simulink model "threeDiskOscillatorRig_Q2_3_v2"  (R2020a)
settings: Solver=VariableStepAuto  StartTime=0.0  StopTime=simTime  RelTol=1e-8
values from neighbouring files (symbols this model uses):
  atan_scale = 100    [ECP_values_final.mat]    (also in Q2-5.mat; Residual_generators.mat; Residual_generatorsQ2.mat; threeDiskOscillator_ALL.m)
  b_1 = 0.00287081256979    [ECP_values_final.mat]    (also in Q2-5.mat; Residual_generators.mat; Residual_generatorsQ2.mat; threeDiskOscillator_ALL.m = mean(ECP_values([6 7])))
  b_2 = 0.000164101446955    [ECP_values_final.mat]    (also in Q2-5.mat; Residual_generators.mat; Residual_generatorsQ2.mat; threeDiskOscillator_ALL.m = mean(ECP_values([8 9])))
  b_3 = 0.000179179608867    [ECP_values_final.mat]    (also in Q2-5.mat; Residual_generators.mat; Residual_generatorsQ2.mat; threeDiskOscillator_ALL.m = mean(ECP_values([10 11])))
  B_change = [1  0; 0  0]    [ECP_values_final.mat]    (also in Q2-5.mat; Residual_generators.mat; Residual_generatorsQ2.mat; threeDiskOscillator_ALL.m = [1 0;0 0])
  C = [1 0 0 0 0 0 0 1 0 0 0 0 ... (18 elements, 3x6)]    [ECP_values_final.mat]    (also in Q2-5.mat; Residual_generators.mat; Residual_generatorsQ2.mat; threeDiskOscillator_ALL.m = double(jacobian(g, x)))
  C_aug = [1 0 0 0 0 0 0 1 0 0 0 0 ... (21 elements, 3x7)]    [ECP_values_final.mat]    (also in Q2-5.mat; Residual_generators.mat; Residual_generatorsQ2.mat; threeDiskOscillator_ALL.m = [C zeros(3, 1)])
  den1 =     [ECP_values_final.mat]    (also in Q2-5.mat; Residual_generators.mat; Residual_generatorsQ2.mat)
  den2 =     [ECP_values_final.mat]    (also in Q2-5.mat; Residual_generators.mat; Residual_generatorsQ2.mat)
  detect_time = 45    [ECP_values_final.mat]    (also in Q2-5.mat = 28.75; Residual_generators.mat = 28.75; Residual_generatorsQ2.mat = 28.75; threeDiskOscillator_ALL.m = 28.75)
  F_aug = [0.990702939697 -4.62811632173 0.0121231655 6.0271208888 2.24543739426e-05 0.0224199828886 0 0.00397798624468 0.985916806084 1.6181632514e-05 0.0121036964897 1.79648757592e-08 ... (49 elements, 7x7)]    [ECP_values_final.mat]    (also in Q2-5.mat; Residual_generators.mat; Residual_generatorsQ2.mat; threeDiskOscillator_ALL.m = [F_d E)
  f_m = [0 -0.025 0]    [ECP_values_final.mat]    (also in Q2-5.mat; Residual_generators.mat; Residual_generatorsQ2.mat; threeDiskOscillator_ALL.m = [0;-0.025;0])
  f_m_time = 8.5    [ECP_values_final.mat]    (also in Q2-5.mat; Residual_generators.mat; Residual_generatorsQ2.mat; threeDiskOscillator_ALL.m)
  f_u = [0 0]    [ECP_values_final.mat]    (also in Q2-5.mat; Residual_generators.mat; Residual_generatorsQ2.mat; threeDiskOscillator_ALL.m = [0;0])
  f_u_time = 25    [ECP_values_final.mat]    (also in Q2-5.mat; Residual_generators.mat; Residual_generatorsQ2.mat; threeDiskOscillator_ALL.m)
  G_aug = [0.00334221577476 1.66717035551 6.79109721451e-06 0.00678170721861 5.02271998836e-09 7.52906281318e-06 0 6.79109721451e-06 0.00678170721861 0.00435611271714 2.16907893788 8.06078126345e-06 ... (14 elements, 7x2)]    [ECP_values_final.mat]    (also in Q2-5.mat; Residual_generators.mat; Residual_generatorsQ2.mat; threeDiskOscillator_ALL.m = [G_d; zeros(1, 2)])
  h = 7.56835261331    [ECP_values_final.mat]    (also in Q2-5.mat; Residual_generators.mat = 0; Residual_generatorsQ2.mat = 0; threeDiskOscillator_ALL.m = chi2inv(1 - P_F, 1)/2)
  J_1 = 0.00238607064451    [ECP_values_final.mat]    (also in Q2-5.mat; Residual_generators.mat; Residual_generatorsQ2.mat; threeDiskOscillator_ALL.m = ECP_values(1))
  J_2 = 0.00182883419357    [ECP_values_final.mat]    (also in Q2-5.mat; Residual_generators.mat; Residual_generatorsQ2.mat; threeDiskOscillator_ALL.m = ECP_values(2))
  J_3 = 0.00182883419357    [ECP_values_final.mat]    (also in Q2-5.mat; Residual_generators.mat; Residual_generatorsQ2.mat; threeDiskOscillator_ALL.m = ECP_values(3))
  k_1 = 2.78736928639    [ECP_values_final.mat]    (also in Q2-5.mat; Residual_generators.mat; Residual_generatorsQ2.mat; threeDiskOscillator_ALL.m = ECP_values(4))
  k_2 = 2.53389832968    [ECP_values_final.mat]    (also in Q2-5.mat; Residual_generators.mat; Residual_generatorsQ2.mat; threeDiskOscillator_ALL.m = ECP_values(5))
  L_aug = [0.925638751325 22.7990667466 0.000933229250844 2.83148520586 4.75495506307e-05 0.155666275776 0.870972503145 0.000933229250844 2.5605224603 0.918032233948 0.967278648673 0.000147626320163 ... (21 elements, 7x3)]    [ECP_values_final.mat]    (also in Q2-5.mat; Residual_generators.mat; Residual_generatorsQ2.mat; threeDiskOscillator_ALL.m = dlqe(F_aug,eye(7),C_aug,1e-3*eye(7),deg2rad(0.0056)*eye(3)))
  num1 =     [ECP_values_final.mat]    (also in Q2-5.mat; Residual_generators.mat; Residual_generatorsQ2.mat)
  num2 =     [ECP_values_final.mat]    (also in Q2-5.mat; Residual_generators.mat; Residual_generatorsQ2.mat)
  r_window = [0 0 0 0 0 0 0 0 0 0 0 0 ... (64 elements, 64x1)]    [ECP_values_final.mat]    (also in Q2-5.mat = [0 0 0 0 0 0 0 0 0 0 0 0 ... (265 elements, 265x1)]; threeDiskOscillator_ALL.m = zeros(M,1); threeDiskOscillator_Q6.m = zeros(floor(M),1); threeDiskOscillator_Q8.m = zeros(floor(M),1))
  sigma_meas = [0.0093  0  0; 0  0.0093  0; 0  0  0.0093]    [ECP_values_final.mat]    (also in Q2-5.mat; Residual_generators.mat; Residual_generatorsQ2.mat; threeDiskOscillator_ALL.m = 0.0093*eye(3))
  T_Cm = 0.0969711017207    [ECP_values_final.mat]    (also in Q2-5.mat; Residual_generators.mat; Residual_generatorsQ2.mat; threeDiskOscillator_ALL.m = ECP_values(13))
  T_Cp = 0.0714454263135    [ECP_values_final.mat]    (also in Q2-5.mat; Residual_generators.mat; Residual_generatorsQ2.mat; threeDiskOscillator_ALL.m = ECP_values(12))
  T_s = 0.004    [ECP_values_final.mat]    (also in Q2-5.mat; Residual_generators.mat; Residual_generatorsQ2.mat; threeDiskOscillator_ALL.m)
  u_fault = 0    [ECP_values_final.mat]    (also in Q2-5.mat; Residual_generators.mat; Residual_generatorsQ2.mat; threeDiskOscillator_ALL.m)
  w_th = 0.75    [ECP_values_final.mat]    (also in Q2-5.mat; Residual_generators.mat; Residual_generatorsQ2.mat; threeDiskOscillator_ALL.m)
  x_0 = [0 0 0 0 0 0]    [ECP_values_final.mat]    (also in Q2-5.mat; Residual_generators.mat; Residual_generatorsQ2.mat; threeDiskOscillator_ALL.m = [0;0;0;0;0;0])
libraries: simulink x1
settings Model: Creator=dimpa  LastModifiedBy=Administrator
settings DataIOCC: ReturnWorkspaceOutputs=off
settings DebuggingCC: ArithmeticOperatorsInVariantConditions=warning
settings SFSimCC: SimUseLocalCustomCode=off  CustomCodeUndefinedFunction=UseInterfaceOnly
settings RTWCC: RTWUseLocalCustomCode=off

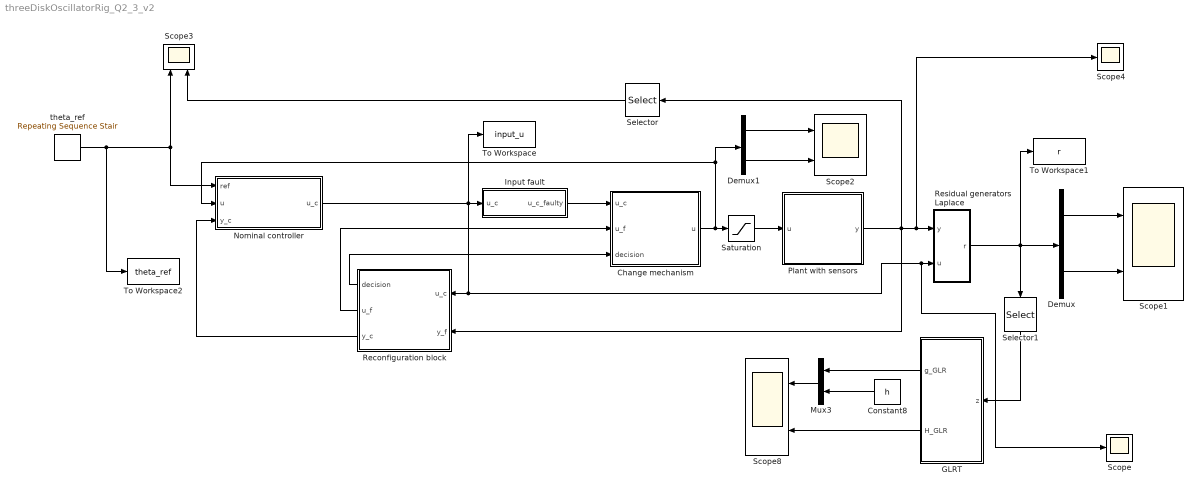
== system threeDiskOscillatorRig_Q2_3_v2 ==
  Change mechanism : Subsystem
  Constant8 : Constant  Value=h
  Demux : Demux  Outputs=2
  Demux1 : Demux  Outputs=2
  GLRT : Subsystem
  Input fault : Subsystem
  Mux3 : Mux  Inputs=2
  Nominal controller : Subsystem
  Plant with sensors : Subsystem
  Reconfiguration block : Subsystem
  Residual generators Laplace : Subsystem
  Saturation : Saturate  UpperLimit=2  LowerLimit=-2
  Scope : Scope
  Scope{1..3,8} (4 alike) : Scope  NumInputPorts=2
  Scope4 : Scope
  Selector : Selector  InputPortWidth=3  IndexOptions=Index vector (dialog)  Indices=[3]  OutputSizes=1
  Selector1 : Selector  InputPortWidth=2  IndexOptions=Index vector (dialog)  Indices=[2]  OutputSizes=1
  To Workspace : ToWorkspace  VariableName=input_u  SaveFormat=Timeseries  SampleTime=T_s
  To Workspace1 : ToWorkspace  VariableName=r  SaveFormat=Timeseries  SampleTime=T_s
  To Workspace2 : ToWorkspace  VariableName=theta_ref  SaveFormat=Timeseries  SampleTime=T_s
  theta_ref : simulink/Sources/Repeating Sequence Stair  OutValues=[0 1.57 0]  tsamp=5  OutMin=[]  OutMax=[]  OutDataTypeStr=double  OutputDataTypeScalingMode=double  OutDataType=fixdt(0,8)  ConRadixGroup=Best Precision: Vector-wise  OutScaling=2^-12
  wires:
  Selector/1 -> Scope3/2
  Saturation/1 -> Plant with sensors/1(u)
  theta_ref/1 -> Nominal controller/1(ref), Scope3/1, To Workspace2/1
  Plant with sensors/1(y) -> Reconfiguration block/2(y_f), Scope4/1, Residual generators Laplace/1(y), Selector/1
  Residual generators Laplace/1(r) -> Selector1/1, Demux/1, To Workspace1/1
  GLRT/1(g_GLR) -> Mux3/1
  GLRT/2(H_GLR) -> Scope8/2
  Constant8/1 -> Mux3/2
  Mux3/1 -> Scope8/1
  Selector1/1 -> GLRT/1(z)
  Demux/1 -> Scope1/1
  Demux/2 -> Scope1/2
  Demux1/1 -> Scope2/1
  Demux1/2 -> Scope2/2
  Nominal controller/1(u_c) -> Input fault/1(u_c), Scope/1, Residual generators Laplace/2(u), Reconfiguration block/1(u_c), To Workspace/1
  Reconfiguration block/3(y_c) -> Nominal controller/3(y_c)
  Change mechanism/1(u) -> Nominal controller/2(u), Demux1/1, Saturation/1
  Input fault/1(u_c_faulty) -> Change mechanism/1(u_c)
  Reconfiguration block/1(decision) -> Change mechanism/3(decision)
  Reconfiguration block/2(u_f) -> Change mechanism/2(u_f)

== system threeDiskOscillatorRig_Q2_3_v2/Change mechanism ==
  u_c : Inport
  u_f : Inport  Port=2
  decision : Inport  Port=3
  Gain2 : Gain  Gain=B_change  Multiplication=Matrix(K*u) (u vector)
  Scope : Scope
  Switch2 : Switch  OutDataTypeStr=double
  u : Outport
  wires:
  Gain2/1 -> Switch2/3
  decision/1 -> Scope/1, Switch2/2
  u_c/1 -> Switch2/1
  Switch2/1 -> u/1
  u_f/1 -> Gain2/1

== system threeDiskOscillatorRig_Q2_3_v2/GLRT ==
  z : Inport
  Delay : Delay  DelayLength=1  InitialCondition=r_window  SampleTime=T_s
  MATLAB Function : MATLAB Function  TreatAsAtomicUnit=on
  g_GLR : Outport  VectorParamsAs1DForOutWhenUnconnected=off
  H_GLR : Outport  Port=2  VectorParamsAs1DForOutWhenUnconnected=off
  wires:
  z/1 -> MATLAB Function/1(r_new)
  MATLAB Function/3(r_window) -> Delay/1
  MATLAB Function/2(g) -> g_GLR/1
  MATLAB Function/1(H) -> H_GLR/1
  Delay/1 -> MATLAB Function/2("r_window ")

== system threeDiskOscillatorRig_Q2_3_v2/Input fault ==
  u_c : Inport
  Sum4 : Sum  Inputs=|++
  f_u : Step  Time=f_u_time  After=f_u  SampleTime=0
  u_c_faulty : Outport
  wires:
  u_c/1 -> Sum4/1
  Sum4/1 -> u_c_faulty/1
  f_u/1 -> Sum4/2

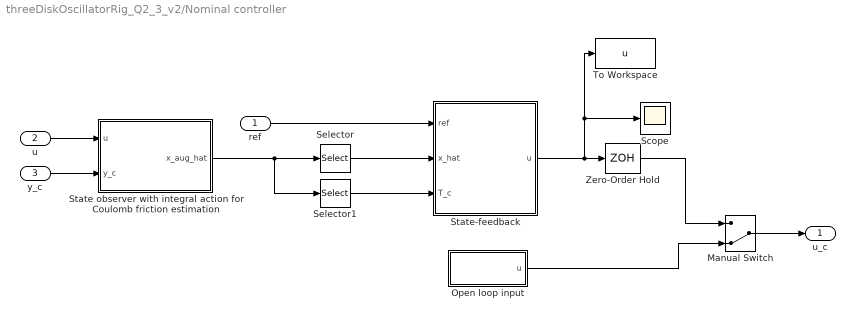
== system threeDiskOscillatorRig_Q2_3_v2/Nominal controller ==
  ref : Inport
  u : Inport  Port=2
  y_c : Inport  Port=3
  Manual Switch : ManualSwitch  CurrentSetting=0
  Open loop input : Subsystem
  Scope : Scope
  Selector : Selector  InputPortWidth=7  IndexOptions=Index vector (dialog)  Indices=[1:6]  OutputSizes=1
  Selector1 : Selector  InputPortWidth=7  IndexOptions=Index vector (dialog)  Indices=[7]  OutputSizes=1
  State observer with integral action for Coulomb friction estimation : Subsystem
  State-feedback : Subsystem
  To Workspace : ToWorkspace  VariableName=u  SaveFormat=Timeseries  SampleTime=T_s
  Zero-Order Hold : ZeroOrderHold  SampleTime=T_s
  u_c : Outport
  wires:
  Zero-Order Hold/1 -> Manual Switch/1
  y_c/1 -> State observer with integral action for Coulomb friction estimation/2(y_c)
  u/1 -> State observer with integral action for Coulomb friction estimation/1(u)
  Open loop input/1(u) -> Manual Switch/2
  Manual Switch/1 -> u_c/1
  Selector/1 -> State-feedback/2(x_hat)
  Selector1/1 -> State-feedback/3(T_c)
  State observer with integral action for Coulomb friction estimation/1(x_aug_hat) -> Selector1/1, Selector/1
  ref/1 -> State-feedback/1(ref)
  State-feedback/1(u) -> To Workspace/1, Scope/1, Zero-Order Hold/1

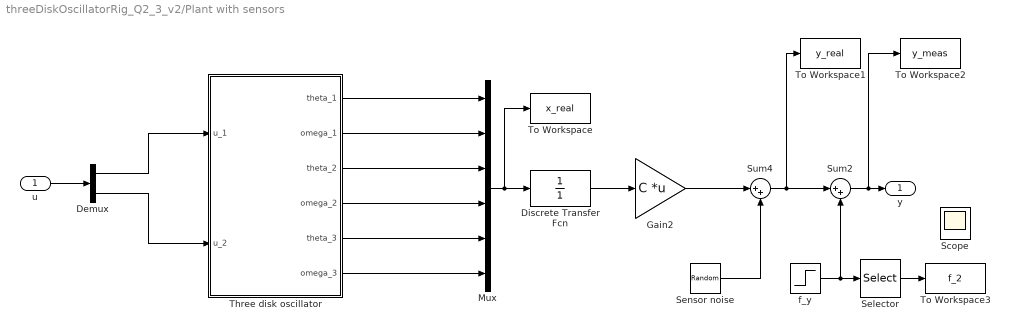
== system threeDiskOscillatorRig_Q2_3_v2/Plant with sensors ==
  u : Inport
  Demux : Demux  Outputs=2
  Discrete Transfer Fcn : DiscreteTransferFcn  Denominator=[1]  SampleTime=T_s
  Gain2 : Gain  Gain=C  Multiplication=Matrix(K*u) (u vector)
  Mux : Mux  Inputs=6
  Scope : Scope
  Selector : Selector  InputPortWidth=3  IndexOptions=Index vector (dialog)  Indices=[2]  OutputSizes=1
  Sensor noise : RandomNumber  Mean=zeros(3,1)  Variance=diag(sigma_meas^2)  SampleTime=T_s
  Sum2 : Sum  Inputs=|++
  Sum4 : Sum  Inputs=|++
  Three disk oscillator : Subsystem
  To Workspace : ToWorkspace  VariableName=x_real  SaveFormat=Timeseries  SampleTime=T_s
  To Workspace1 : ToWorkspace  VariableName=y_real  SaveFormat=Timeseries  SampleTime=T_s
  To Workspace2 : ToWorkspace  VariableName=y_meas  SaveFormat=Timeseries  SampleTime=T_s
  To Workspace3 : ToWorkspace  VariableName=f_2  SaveFormat=Timeseries  SampleTime=T_s
  f_y : Step  Time=f_m_time  Before=[0;0;0]  After=f_m  SampleTime=0
  y : Outport  VectorParamsAs1DForOutWhenUnconnected=off
  wires:
  u/1 -> Demux/1
  Three disk oscillator/2(omega_1) -> Mux/2
  Three disk oscillator/1(theta_1) -> Mux/1
  Mux/1 -> To Workspace/1, Discrete Transfer Fcn/1
  Three disk oscillator/4(omega_2) -> Mux/4
  Three disk oscillator/3(theta_2) -> Mux/3
  Discrete Transfer Fcn/1 -> Gain2/1
  Gain2/1 -> Sum4/1
  Sum4/1 -> To Workspace1/1, Sum2/1
  Three disk oscillator/6(omega_3) -> Mux/6
  Three disk oscillator/5(theta_3) -> Mux/5
  f_y/1 -> Sum2/2, Selector/1
  Sum2/1 -> To Workspace2/1, y/1
  Selector/1 -> To Workspace3/1
  Demux/1 -> Three disk oscillator/1(u_1)
  Demux/2 -> Three disk oscillator/2(u_2)
  Sensor noise/1 -> Sum4/2

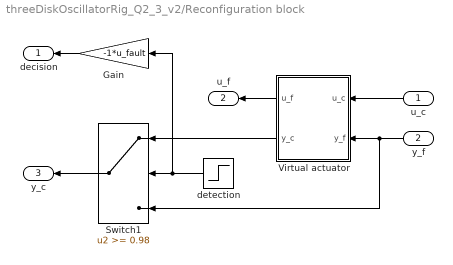
== system threeDiskOscillatorRig_Q2_3_v2/Reconfiguration block ==
  u_c : Inport
  y_f : Inport  Port=2
  Gain : Gain  Gain=-1*u_fault
  Switch1 : Switch  Threshold=0.98
  Virtual actuator : Subsystem
  detection : Step  Time=detect_time  SampleTime=T_s
  decision : Outport  VectorParamsAs1DForOutWhenUnconnected=off
  u_f : Outport  Port=2  VectorParamsAs1DForOutWhenUnconnected=off
  y_c : Outport  Port=3  VectorParamsAs1DForOutWhenUnconnected=off
  wires:
  u_c/1 -> Virtual actuator/1(u_c)
  detection/1 -> Gain/1, Switch1/2
  Switch1/1 -> y_c/1
  Virtual actuator/2(y_c) -> Switch1/1
  y_f/1 -> Virtual actuator/2(y_f), Switch1/3
  Virtual actuator/1(u_f) -> u_f/1
  Gain/1 -> decision/1

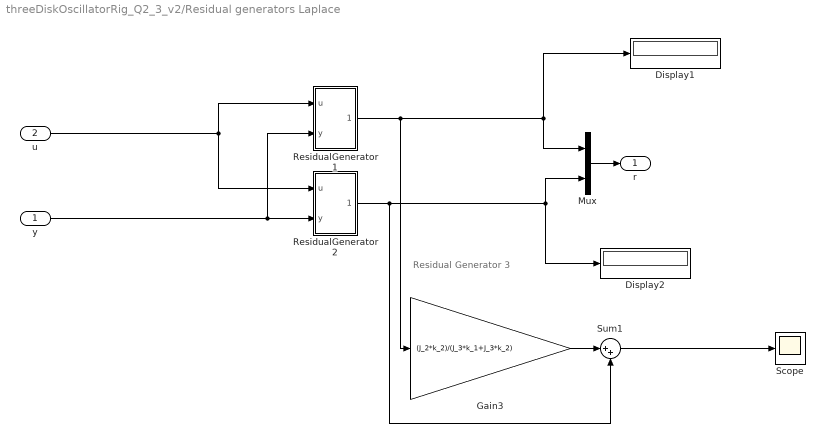
== system threeDiskOscillatorRig_Q2_3_v2/Residual generators Laplace ==
  note: Residual Generator 3
  y : Inport
  u : Inport  Port=2
  Display1 : Display
  Display2 : Display
  Gain3 : Gain  Gain=(J_2*k_2)/(J_3*k_1+J_3*k_2)
  Mux : Mux  Inputs=2
  ResidualGenerator 1 : Subsystem
  ResidualGenerator 2 : Subsystem
  Scope : Scope
  Sum1 : Sum  Inputs=|++
  r : Outport  VectorParamsAs1DForOutWhenUnconnected=off
  wires:
  Mux/1 -> r/1
  u/1 -> ResidualGenerator 2/1(u), ResidualGenerator 1/1(u)
  y/1 -> ResidualGenerator 1/2(y), ResidualGenerator 2/2(y)
  ResidualGenerator 2/1(Out1) -> Mux/2, Display2/1, Sum1/2
  Sum1/1 -> Scope/1
  Gain3/1 -> Sum1/1
  ResidualGenerator 1/1(Out1) -> Display1/1, Mux/1, Gain3/1

== system threeDiskOscillatorRig_Q2_3_v2/Nominal controller/Open loop input ==
  Constant : Constant  Value=3
  Constant1 : Constant  Value=0
  Multiport Switch : MultiPortSwitch
  Mux : Mux  Inputs=2
  Mux1 : Mux  Inputs=2
  Mux2 : Mux  Inputs=2
  Pulse Generator : DiscretePulseGenerator  PulseType=Time based  Period=10  PulseWidth=5
  u : Outport
  wires:
  Constant1/1 -> Mux1/1, Mux/2
  Pulse Generator/1 -> Mux2/2, Mux2/1, Mux1/2, Mux/1
  Constant/1 -> Multiport Switch/1
  Mux2/1 -> Multiport Switch/4
  Mux/1 -> Multiport Switch/2
  Multiport Switch/1 -> u/1
  Mux1/1 -> Multiport Switch/3

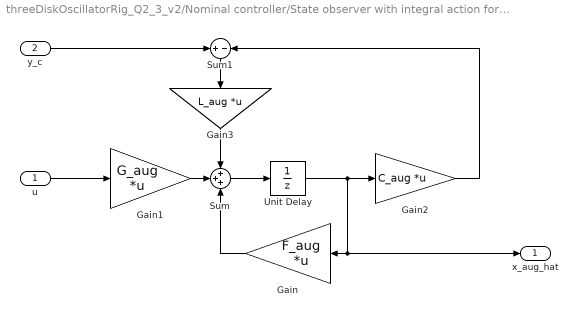
== system threeDiskOscillatorRig_Q2_3_v2/Nominal controller/State observer with integral action for Coulomb friction estimation ==
  u : Inport
  y_c : Inport  Port=2
  Gain : Gain  Gain=F_aug  Multiplication=Matrix(K*u) (u vector)
  Gain1 : Gain  Gain=G_aug  Multiplication=Matrix(K*u) (u vector)
  Gain2 : Gain  Gain=C_aug  Multiplication=Matrix(K*u) (u vector)
  Gain3 : Gain  Gain=L_aug  Multiplication=Matrix(K*u) (u vector)
  Sum : Sum  Inputs=+++
  Sum1 : Sum  Inputs=+-
  Unit Delay : UnitDelay  SampleTime=T_s  HasFrameUpgradeWarning=on
  x_aug_hat : Outport  VectorParamsAs1DForOutWhenUnconnected=off
  wires:
  Unit Delay/1 -> x_aug_hat/1, Gain/1, Gain2/1
  y_c/1 -> Sum1/1
  Sum1/1 -> Gain3/1
  Sum/1 -> Unit Delay/1
  Gain2/1 -> Sum1/2
  u/1 -> Gain1/1
  Gain1/1 -> Sum/2
  Gain/1 -> Sum/3
  Gain3/1 -> Sum/1

== system threeDiskOscillatorRig_Q2_3_v2/Nominal controller/State-feedback ==
  note: Feed-forward term for Coulomb friction
  ref : Inport
  x_hat : Inport  Port=2
  T_c : Inport  Port=3
  Gain2 : Gain  Gain=[1;0]
  State feedback controller : Subsystem
  Sum2 : Sum  Inputs=|+-
  u : Outport  VectorParamsAs1DForOutWhenUnconnected=off
  wires:
  T_c/1 -> Gain2/1
  Gain2/1 -> Sum2/2
  Sum2/1 -> u/1
  ref/1 -> State feedback controller/1(ref)
  x_hat/1 -> State feedback controller/2(x_hat)
  State feedback controller/1(u_fb) -> Sum2/1

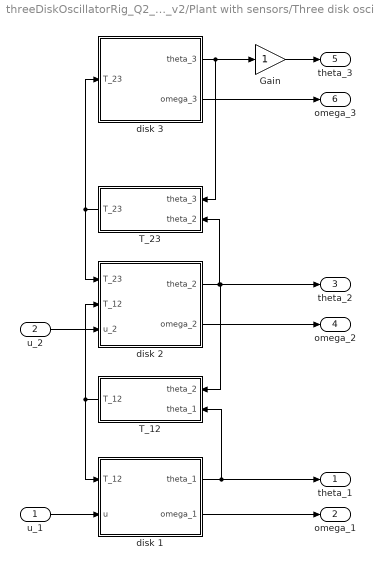
== system threeDiskOscillatorRig_Q2_3_v2/Plant with sensors/Three disk oscillator ==
  u_1 : Inport
  u_2 : Inport  Port=2
  Gain : Gain
  T_12 : Subsystem
  T_23 : Subsystem
  disk 1 : Subsystem
  disk 2 : Subsystem
  disk 3 : Subsystem
  theta_1 : Outport  VectorParamsAs1DForOutWhenUnconnected=off
  omega_1 : Outport  Port=2  VectorParamsAs1DForOutWhenUnconnected=off
  theta_2 : Outport  Port=3  VectorParamsAs1DForOutWhenUnconnected=off
  omega_2 : Outport  Port=4  VectorParamsAs1DForOutWhenUnconnected=off
  theta_3 : Outport  Port=5  VectorParamsAs1DForOutWhenUnconnected=off
  omega_3 : Outport  Port=6  VectorParamsAs1DForOutWhenUnconnected=off
  wires:
  T_23/1(T_23) -> disk 2/1(T_23), disk 3/1(T_23)
  disk 1/1(theta_1) -> T_12/2(theta_1), theta_1/1
  disk 2/1(theta_2) -> T_23/2(theta_2), theta_2/1, T_12/1(theta_2)
  T_12/1(T_12) -> disk 1/1(T_12), disk 2/2(T_12)
  disk 3/2(omega_3) -> omega_3/1
  disk 1/2(omega_1) -> omega_1/1
  disk 2/2(omega_2) -> omega_2/1
  u_1/1 -> disk 1/2(u)
  disk 3/1(theta_3) -> Gain/1, T_23/1(theta_3)
  Gain/1 -> theta_3/1
  u_2/1 -> disk 2/3(u_2)

== system threeDiskOscillatorRig_Q2_3_v2/Reconfiguration block/Virtual actuator ==
  u_c : Inport
  y_f : Inport  Port=2
  u_f : Outport  VectorParamsAs1DForOutWhenUnconnected=off
  y_c : Outport  Port=2  VectorParamsAs1DForOutWhenUnconnected=off

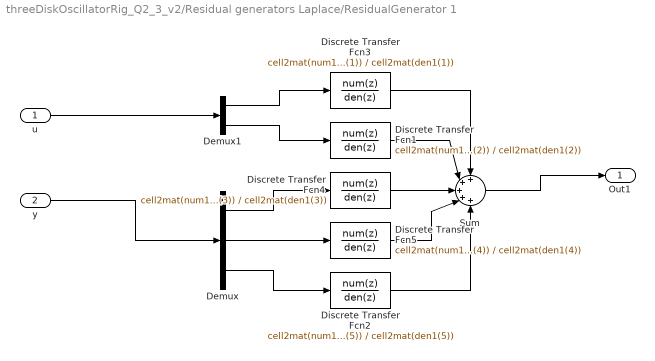
== system threeDiskOscillatorRig_Q2_3_v2/Residual generators Laplace/ResidualGenerator 1 ==
  u : Inport
  y : Inport  Port=2
  Demux : Demux  Outputs=3
  Demux1 : Demux  Outputs=2
  Discrete Transfer Fcn1 : DiscreteTransferFcn  Numerator=cell2mat(num1(2))  Denominator=cell2mat(den1(2))
  Discrete Transfer Fcn2 : DiscreteTransferFcn  Numerator=cell2mat(num1(5))  Denominator=cell2mat(den1(5))
  Discrete Transfer Fcn3 : DiscreteTransferFcn  Numerator=cell2mat(num1(1))  Denominator=cell2mat(den1(1))
  Discrete Transfer Fcn4 : DiscreteTransferFcn  Numerator=cell2mat(num1(3))  Denominator=cell2mat(den1(3))
  Discrete Transfer Fcn5 : DiscreteTransferFcn  Numerator=cell2mat(num1(4))  Denominator=cell2mat(den1(4))
  Sum : Sum  Inputs=+++++
  Out1 : Outport
  wires:
  Demux/2 -> Discrete Transfer Fcn5/1
  Discrete Transfer Fcn5/1 -> Sum/4
  Sum/1 -> Out1/1
  Discrete Transfer Fcn3/1 -> Sum/1
  Demux/1 -> Discrete Transfer Fcn4/1
  Demux/3 -> Discrete Transfer Fcn2/1
  Discrete Transfer Fcn1/1 -> Sum/2
  Discrete Transfer Fcn4/1 -> Sum/3
  Demux1/1 -> Discrete Transfer Fcn3/1
  Demux1/2 -> Discrete Transfer Fcn1/1
  Discrete Transfer Fcn2/1 -> Sum/5
  y/1 -> Demux/1
  u/1 -> Demux1/1

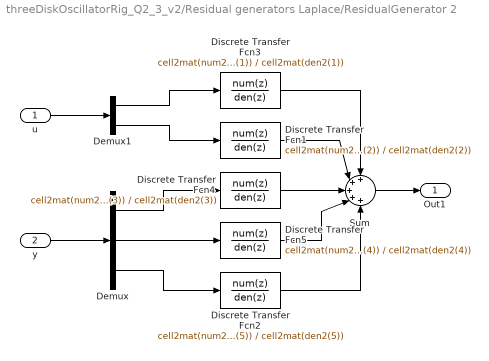
== system threeDiskOscillatorRig_Q2_3_v2/Residual generators Laplace/ResidualGenerator 2 ==
  u : Inport
  y : Inport  Port=2
  Demux : Demux  Outputs=3
  Demux1 : Demux  Outputs=2
  Discrete Transfer Fcn1 : DiscreteTransferFcn  Numerator=cell2mat(num2(2))  Denominator=cell2mat(den2(2))
  Discrete Transfer Fcn2 : DiscreteTransferFcn  Numerator=cell2mat(num2(5))  Denominator=cell2mat(den2(5))
  Discrete Transfer Fcn3 : DiscreteTransferFcn  Numerator=cell2mat(num2(1))  Denominator=cell2mat(den2(1))
  Discrete Transfer Fcn4 : DiscreteTransferFcn  Numerator=cell2mat(num2(3))  Denominator=cell2mat(den2(3))
  Discrete Transfer Fcn5 : DiscreteTransferFcn  Numerator=cell2mat(num2(4))  Denominator=cell2mat(den2(4))
  Sum : Sum  Inputs=+++++
  Out1 : Outport
  wires:
  Demux/2 -> Discrete Transfer Fcn5/1
  Discrete Transfer Fcn5/1 -> Sum/4
  Sum/1 -> Out1/1
  Discrete Transfer Fcn3/1 -> Sum/1
  Demux/1 -> Discrete Transfer Fcn4/1
  Demux/3 -> Discrete Transfer Fcn2/1
  Discrete Transfer Fcn1/1 -> Sum/2
  Discrete Transfer Fcn4/1 -> Sum/3
  Demux1/1 -> Discrete Transfer Fcn3/1
  Demux1/2 -> Discrete Transfer Fcn1/1
  Discrete Transfer Fcn2/1 -> Sum/5
  y/1 -> Demux/1
  u/1 -> Demux1/1

== system threeDiskOscillatorRig_Q2_3_v2/Nominal controller/State-feedback/State feedback controller ==
  ref : Inport
  x_hat : Inport  Port=2
  u_fb : Outport

== system threeDiskOscillatorRig_Q2_3_v2/Plant with sensors/Three disk oscillator/T_12 ==
  theta_2 : Inport
  theta_1 : Inport  Port=2
  Gain : Gain  Gain=k_1
  Sum : Sum  Inputs=|+-
  T_12 : Outport  VectorParamsAs1DForOutWhenUnconnected=off
  wires:
  theta_2/1 -> Sum/2
  theta_1/1 -> Sum/1
  Sum/1 -> Gain/1
  Gain/1 -> T_12/1

== system threeDiskOscillatorRig_Q2_3_v2/Plant with sensors/Three disk oscillator/T_23 ==
  theta_3 : Inport
  theta_2 : Inport  Port=2
  Gain : Gain  Gain=k_2
  Sum : Sum  Inputs=-+|
  T_23 : Outport  VectorParamsAs1DForOutWhenUnconnected=off
  wires:
  Gain/1 -> T_23/1
  Sum/1 -> Gain/1
  theta_3/1 -> Sum/1
  theta_2/1 -> Sum/2

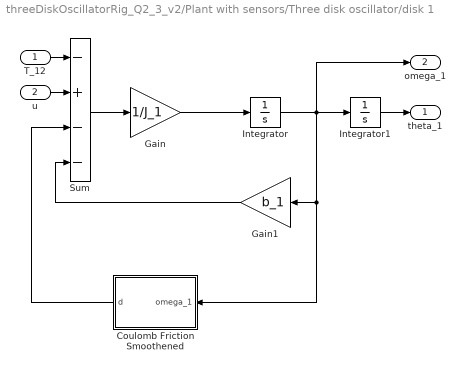
== system threeDiskOscillatorRig_Q2_3_v2/Plant with sensors/Three disk oscillator/disk 1 ==
  T_12 : Inport
  u : Inport  Port=2
  Coulomb Friction Smoothened : Subsystem
  Gain : Gain  Gain=1/J_1
  Gain1 : Gain  Gain=b_1
  Integrator : Integrator  InitialCondition=x_0(2)
  Integrator1 : Integrator  InitialCondition=x_0(1)
  Sum : Sum  Inputs=-+--
  theta_1 : Outport  VectorParamsAs1DForOutWhenUnconnected=off
  omega_1 : Outport  Port=2  VectorParamsAs1DForOutWhenUnconnected=off
  wires:
  Sum/1 -> Gain/1
  Integrator/1 -> Integrator1/1, omega_1/1, Coulomb Friction Smoothened/1(omega_1), Gain1/1
  Gain1/1 -> Sum/4
  Integrator1/1 -> theta_1/1
  T_12/1 -> Sum/1
  u/1 -> Sum/2
  Gain/1 -> Integrator/1
  Coulomb Friction Smoothened/1(d) -> Sum/3

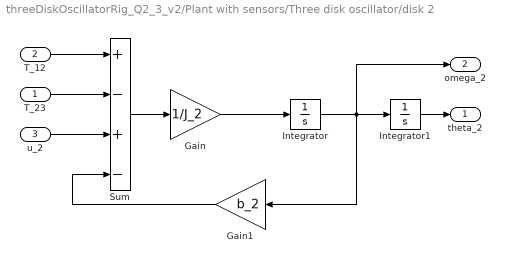
== system threeDiskOscillatorRig_Q2_3_v2/Plant with sensors/Three disk oscillator/disk 2 ==
  T_23 : Inport
  T_12 : Inport  Port=2
  u_2 : Inport  Port=3
  Gain : Gain  Gain=1/J_2
  Gain1 : Gain  Gain=b_2
  Integrator : Integrator  InitialCondition=x_0(4)
  Integrator1 : Integrator  InitialCondition=x_0(3)
  Sum : Sum  Inputs=+-+-
  theta_2 : Outport  VectorParamsAs1DForOutWhenUnconnected=off
  omega_2 : Outport  Port=2  VectorParamsAs1DForOutWhenUnconnected=off
  wires:
  T_23/1 -> Sum/2
  T_12/1 -> Sum/1
  Integrator1/1 -> theta_2/1
  Gain1/1 -> Sum/4
  Gain/1 -> Integrator/1
  Integrator/1 -> Integrator1/1, Gain1/1, omega_2/1
  Sum/1 -> Gain/1
  u_2/1 -> Sum/3

== system threeDiskOscillatorRig_Q2_3_v2/Plant with sensors/Three disk oscillator/disk 3 ==
  T_23 : Inport
  Gain : Gain  Gain=1/J_3
  Gain1 : Gain  Gain=b_3
  Integrator : Integrator  InitialCondition=x_0(6)
  Integrator1 : Integrator  InitialCondition=x_0(5)
  Sum : Sum  Inputs=|+-
  theta_3 : Outport  VectorParamsAs1DForOutWhenUnconnected=off
  omega_3 : Outport  Port=2  VectorParamsAs1DForOutWhenUnconnected=off
  wires:
  Sum/1 -> Gain/1
  Integrator/1 -> Integrator1/1, omega_3/1, Gain1/1
  Gain/1 -> Integrator/1
  Gain1/1 -> Sum/2
  Integrator1/1 -> theta_3/1
  T_23/1 -> Sum/1

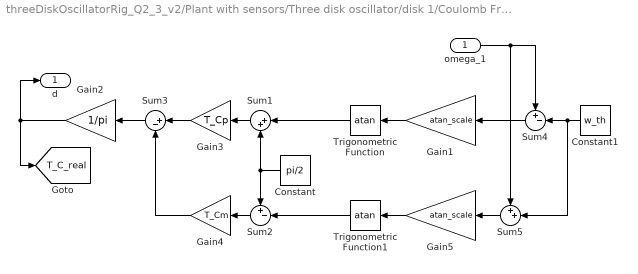
== system threeDiskOscillatorRig_Q2_3_v2/Plant with sensors/Three disk oscillator/disk 1/Coulomb Friction Smoothened ==
  omega_1 : Inport
  Constant : Constant  Value=pi/2
  Constant1 : Constant  Value=w_th
  Gain1 : Gain  Gain=atan_scale
  Gain2 : Gain  Gain=1/pi
  Gain3 : Gain  Gain=T_Cp
  Gain4 : Gain  Gain=T_Cm
  Gain5 : Gain  Gain=atan_scale
  Sum1 : Sum  Inputs=|++
  Sum2 : Sum  Inputs=+-|
  Sum3 : Sum  Inputs=|+-
  Sum4 : Sum  Inputs=+-|
  Sum5 : Sum  Inputs=++|
  Trigonometric Function : Trigonometry  Operator=atan
  Trigonometric Function1 : Trigonometry  Operator=atan
  d : Outport  VectorParamsAs1DForOutWhenUnconnected=off
  tag scope: T_C_real=global
  wires:
  Gain1/1 -> Trigonometric Function/1
  Sum1/1 -> Gain3/1
  Constant/1 -> Sum2/1, Sum1/2
  Sum2/1 -> Gain4/1
  Sum3/1 -> Gain2/1
  Trigonometric Function/1 -> Sum1/1
  Gain4/1 -> Sum3/2
  Gain2/1 -> [T_C_real], d/1
  omega_1/1 -> Sum5/1, Sum4/1
  Gain3/1 -> Sum3/1
  Sum4/1 -> Gain1/1
  Constant1/1 -> Sum5/2, Sum4/2
  Gain5/1 -> Trigonometric Function1/1
  Sum5/1 -> Gain5/1
  Trigonometric Function1/1 -> Sum2/2

== matlab function threeDiskOscillatorRig_Q2_3_v2/GLRT/MATLAB Function ==
  data: r_new input; H output; r_window input; g output; r_window output
function [H, g, r_window] = GLR(r_new, r_window)

sigma = 0.36229693539067544172329302373852;
mu_0 = 0;
M = 265;
h=7.5684;

r_window = [r_window(2:end); r_new];


%Using equation 7.35 from the book

%calculating g from a running window.
g = 1/(2*sigma^2*M)*max(sum(r_window-mu_0))^2;

if (g > h)
    H = 1;
else
    H = 0;
end
